simulink model "Suspension_shaker_rig_model"  (R2024b)
settings: Solver=VariableStepAuto  StartTime=0.0  StopTime=10  RelTol=1e-3
values from neighbouring files (symbols this model uses):
  a = 1.8    [Suspension_shaker_rig_model_parameters.m]
  A = 1.25    [Suspension_shaker_rig_model_parameters.m]
  a1f = -1e-5    (= -1e-05)    [Suspension_shaker_rig_model_parameters.m]
  a2f = 0.95    [Suspension_shaker_rig_model_parameters.m]
  b = L-a    (= 1.7)    [Suspension_shaker_rig_model_parameters.m]
  Bf = 0.0813    [Suspension_shaker_rig_model_parameters.m]
  Br = 0.0925    [Suspension_shaker_rig_model_parameters.m]
  cdf = 1400    [Suspension_shaker_rig_model_parameters.m]
  cdr = 1800    [Suspension_shaker_rig_model_parameters.m]
  Cf = 1.2947    [Suspension_shaker_rig_model_parameters.m]
  Cr = 1.2617    [Suspension_shaker_rig_model_parameters.m]
  Cz = 1.0    (= 1)    [Suspension_shaker_rig_model_parameters.m]
  Ef = -8.3966    [Suspension_shaker_rig_model_parameters.m]
  Er = -8.7012    [Suspension_shaker_rig_model_parameters.m]
  g = 9.81    [Suspension_shaker_rig_model_parameters.m]
  hrcf = 0.04    [Suspension_shaker_rig_model_parameters.m]
  hrcr = 0.06    [Suspension_shaker_rig_model_parameters.m]
  husmf = r    (= 0.375)    [Suspension_shaker_rig_model_parameters.m]
  husmr = r    (= 0.375)    [Suspension_shaker_rig_model_parameters.m]
  I = 3500    [Suspension_shaker_rig_model_parameters.m]
  Ixx = 300    [Suspension_shaker_rig_model_parameters.m]
  Iyy = 1350    [Suspension_shaker_rig_model_parameters.m]
  karbf = 5000    [Suspension_shaker_rig_model_parameters.m]
  karbr = 1000    [Suspension_shaker_rig_model_parameters.m]
  ksf = 67500    [Suspension_shaker_rig_model_parameters.m]
  ksr = 100000    [Suspension_shaker_rig_model_parameters.m]
  ktyre = 400000    [Suspension_shaker_rig_model_parameters.m]
  L = 3.5    [Suspension_shaker_rig_model_parameters.m]
  m = 850    [Suspension_shaker_rig_model_parameters.m]
  ms = m-(musf+musr)    (= 817.5)    [Suspension_shaker_rig_model_parameters.m]
  musf = 15.00    (= 15)    [Suspension_shaker_rig_model_parameters.m]
  musr = 17.50    (= 17.5)    [Suspension_shaker_rig_model_parameters.m]
  rho = 1.225    [Suspension_shaker_rig_model_parameters.m]
  tr = 1.85    [Suspension_shaker_rig_model_parameters.m]
  z0tfl = (0.5*ms*b/L+musf)*g/ktyre    (= 0.00523696339286)    [Suspension_shaker_rig_model_parameters.m]
  z0tfr = (0.5*ms*b/L+musf)*g/ktyre    (= 0.00523696339286)    [Suspension_shaker_rig_model_parameters.m]
  z0trl = (0.5*ms*a/L+musr)*g/ktyre    (= 0.00558469285714)    [Suspension_shaker_rig_model_parameters.m]
  z0trr = (0.5*ms*a/L+musr)*g/ktyre    (= 0.00558469285714)    [Suspension_shaker_rig_model_parameters.m]
libraries: aerolibconvert2 x5
settings Model: Creator=jayku  LastModifiedBy=jayku

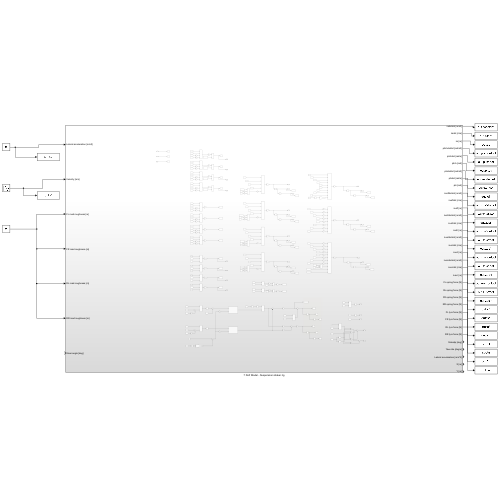
[thumbnail: Simulink's stored preview of the top-level diagram]
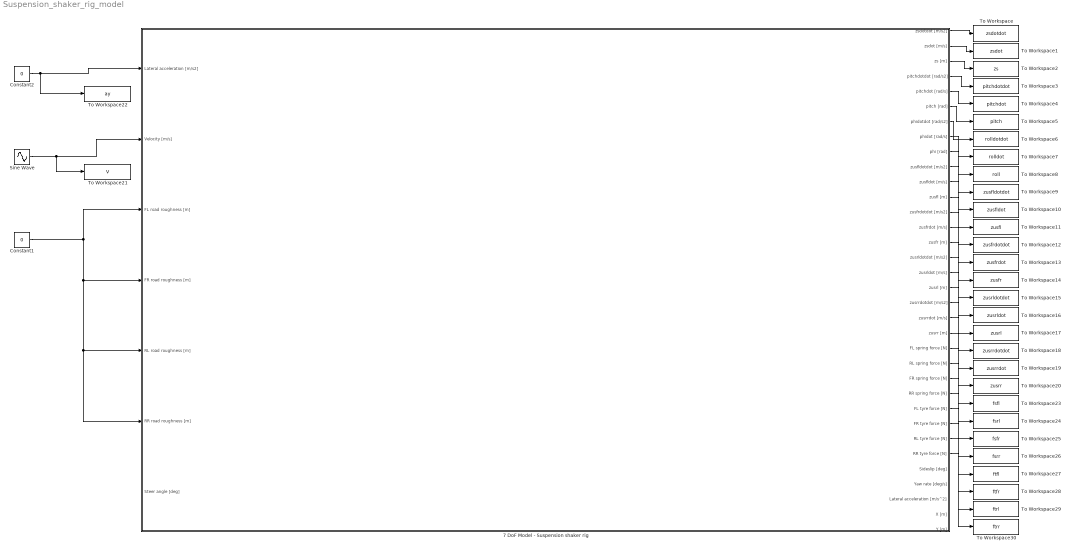
== system Suspension_shaker_rig_model ==
  7 DoF Model - Suspension shaker rig : Subsystem
  Constant1 : Constant  Value=0
  Constant2 : Constant  Value=0
  Sine Wave : Sin  Amplitude=0.01  Frequency=2*pi*1  SampleTime=0
  To Workspace : ToWorkspace  VariableName=zsdotdot  SaveFormat=Timeseries  SampleTime=-1
  To Workspace1 : ToWorkspace  VariableName=zsdot  SaveFormat=Timeseries  SampleTime=-1
  To Workspace10 : ToWorkspace  VariableName=zusfldot  SaveFormat=Timeseries  SampleTime=-1
  To Workspace11 : ToWorkspace  VariableName=zusfl  SaveFormat=Timeseries  SampleTime=-1
  To Workspace12 : ToWorkspace  VariableName=zusfrdotdot  SaveFormat=Timeseries  SampleTime=-1
  To Workspace13 : ToWorkspace  VariableName=zusfrdot  SaveFormat=Timeseries  SampleTime=-1
  To Workspace14 : ToWorkspace  VariableName=zusfr  SaveFormat=Timeseries  SampleTime=-1
  To Workspace15 : ToWorkspace  VariableName=zusrldotdot  SaveFormat=Timeseries  SampleTime=-1
  To Workspace16 : ToWorkspace  VariableName=zusrldot  SaveFormat=Timeseries  SampleTime=-1
  To Workspace17 : ToWorkspace  VariableName=zusrl  SaveFormat=Timeseries  SampleTime=-1
  To Workspace18 : ToWorkspace  VariableName=zusrrdotdot  SaveFormat=Timeseries  SampleTime=-1
  To Workspace19 : ToWorkspace  VariableName=zusrrdot  SaveFormat=Timeseries  SampleTime=-1
  To Workspace2 : ToWorkspace  VariableName=zs  SaveFormat=Timeseries  SampleTime=-1
  To Workspace20 : ToWorkspace  VariableName=zusrr  SaveFormat=Timeseries  SampleTime=-1
  To Workspace21 : ToWorkspace  VariableName=V  SaveFormat=Timeseries  SampleTime=-1
  To Workspace22 : ToWorkspace  VariableName=ay  SaveFormat=Timeseries  SampleTime=-1
  To Workspace23 : ToWorkspace  VariableName=fsfl  SaveFormat=Timeseries  SampleTime=-1
  To Workspace24 : ToWorkspace  VariableName=fsrl  SaveFormat=Timeseries  SampleTime=-1
  To Workspace25 : ToWorkspace  VariableName=fsfr  SaveFormat=Timeseries  SampleTime=-1
  To Workspace26 : ToWorkspace  VariableName=fsrr  SaveFormat=Timeseries  SampleTime=-1
  To Workspace27 : ToWorkspace  VariableName=ftfl  SaveFormat=Timeseries  SampleTime=-1
  To Workspace28 : ToWorkspace  VariableName=ftfr  SaveFormat=Timeseries  SampleTime=-1
  To Workspace29 : ToWorkspace  VariableName=ftrl  SaveFormat=Timeseries  SampleTime=-1
  To Workspace3 : ToWorkspace  VariableName=pitchdotdot  SaveFormat=Timeseries  SampleTime=-1
  To Workspace30 : ToWorkspace  VariableName=ftrr  SaveFormat=Timeseries  SampleTime=-1
  To Workspace4 : ToWorkspace  VariableName=pitchdot  SaveFormat=Timeseries  SampleTime=-1
  To Workspace5 : ToWorkspace  VariableName=pitch  SaveFormat=Timeseries  SampleTime=-1
  To Workspace6 : ToWorkspace  VariableName=rolldotdot  SaveFormat=Timeseries  SampleTime=-1
  To Workspace7 : ToWorkspace  VariableName=rolldot  SaveFormat=Timeseries  SampleTime=-1
  To Workspace8 : ToWorkspace  VariableName=roll  SaveFormat=Timeseries  SampleTime=-1
  To Workspace9 : ToWorkspace  VariableName=zusfldotdot  SaveFormat=Timeseries  SampleTime=-1
  wires:
  7 DoF Model - Suspension shaker rig/1(zsdotdot [m/s2]) -> To Workspace/1
  7 DoF Model - Suspension shaker rig/2(zsdot [m/s]) -> To Workspace1/1
  7 DoF Model - Suspension shaker rig/3(zs [m]) -> To Workspace2/1
  7 DoF Model - Suspension shaker rig/4(pitchdotdot [rad/s2]) -> To Workspace3/1
  7 DoF Model - Suspension shaker rig/5(pitchdot [rad/s]) -> To Workspace4/1
  7 DoF Model - Suspension shaker rig/6(pitch [rad]) -> To Workspace5/1
  7 DoF Model - Suspension shaker rig/7(phidotdot [rad/s2]) -> To Workspace6/1
  7 DoF Model - Suspension shaker rig/8(phidot [rad/s]) -> To Workspace7/1
  7 DoF Model - Suspension shaker rig/9(phi [rad]) -> To Workspace8/1
  7 DoF Model - Suspension shaker rig/10(zusfldotdot [m/s2]) -> To Workspace9/1
  7 DoF Model - Suspension shaker rig/11(zusfldot [m/s]) -> To Workspace10/1
  7 DoF Model - Suspension shaker rig/12(zusfl [m]) -> To Workspace11/1
  7 DoF Model - Suspension shaker rig/13(zusfrdotdot [m/s2]) -> To Workspace12/1
  7 DoF Model - Suspension shaker rig/14(zusfrdot [m/s]) -> To Workspace13/1
  7 DoF Model - Suspension shaker rig/15(zusfr [m]) -> To Workspace14/1
  7 DoF Model - Suspension shaker rig/16(zusrldotdot [m/s2]) -> To Workspace15/1
  7 DoF Model - Suspension shaker rig/17(zusrldot [m/s]) -> To Workspace16/1
  7 DoF Model - Suspension shaker rig/18(zusrl [m]) -> To Workspace17/1
  7 DoF Model - Suspension shaker rig/19(zusrrdotdot [m/s2]) -> To Workspace18/1
  7 DoF Model - Suspension shaker rig/20(zusrrdot [m/s]) -> To Workspace19/1
  7 DoF Model - Suspension shaker rig/21(zusrr [m]) -> To Workspace20/1
  Constant2/1 -> 7 DoF Model - Suspension shaker rig/1(Lateral acceleration [m/s2]), To Workspace22/1
  Sine Wave/1 -> 7 DoF Model - Suspension shaker rig/2(Velocity [m/s]), To Workspace21/1
  7 DoF Model - Suspension shaker rig/22(FL spring force [N]) -> To Workspace23/1
  7 DoF Model - Suspension shaker rig/23(RL spring force [N]) -> To Workspace24/1
  7 DoF Model - Suspension shaker rig/24(FR spring force [N]) -> To Workspace25/1
  7 DoF Model - Suspension shaker rig/25(RR spring force [N]) -> To Workspace26/1
  7 DoF Model - Suspension shaker rig/26(FL tyre force [N]) -> To Workspace27/1
  7 DoF Model - Suspension shaker rig/27(FR tyre force [N]) -> To Workspace28/1
  7 DoF Model - Suspension shaker rig/28(RL tyre force [N]) -> To Workspace29/1
  7 DoF Model - Suspension shaker rig/29(RR tyre force [N]) -> To Workspace30/1
  Constant1/1 -> 7 DoF Model - Suspension shaker rig/5(RL road roughness [m]), 7 DoF Model - Suspension shaker rig/6(RR road roughness [m]), 7 DoF Model - Suspension shaker rig/4(FR road roughness [m]), 7 DoF Model - Suspension shaker rig/3(FL road roughness [m])

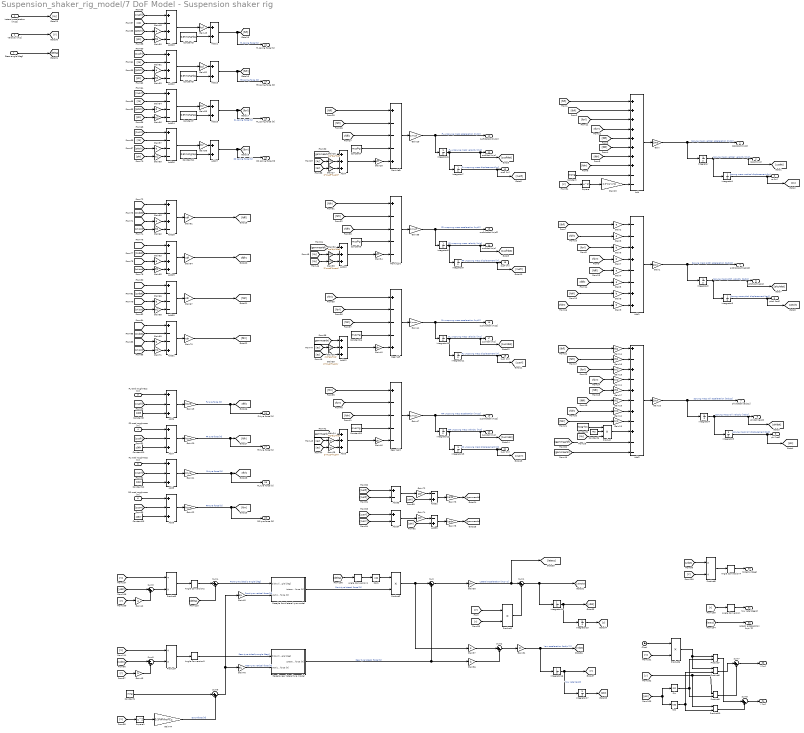
== system Suspension_shaker_rig_model/7 DoF Model - Suspension shaker rig ==
  Lateral acceleration [m/s2] : Inport
  Velocity [m/s] : Inport  Port=2
  FL road roughness [m] : Inport  Port=3
  FR road roughness [m] : Inport  Port=4
  RL road roughness [m] : Inport  Port=5
  RR road roughness [m] : Inport  Port=6
  Steer angle [deg] : Inport  Port=7
  Add : Sum  Inputs=++++++++--
  Add1 : Sum  Inputs=--++--++
  Add{3..4,10,12} (4 alike) : Sum  Inputs=+++
  Add2 : Sum  Inputs=+-+-+-+-+--
  Add20 : Sum  Inputs=+-+-
  Add{21,23,25,27} (4 alike) : Sum
  Add22 : Sum  Inputs=+-+-
  Add24 : Sum  Inputs=+---
  Add26 : Sum  Inputs=+---
  Add28 : Sum  Inputs=+-+-
  Add29 : Sum  Inputs=+-++
  Add30 : Sum  Inputs=+---
  Add31 : Sum  Inputs=+--+
  Add32 : Sum  Inputs=-+
  Add33 : Sum  Inputs=+-
  Add34 : Sum  Inputs=+-
  Add35 : Sum  Inputs=-+
  Add{6..9} (4 alike) : Sum  Inputs=+-+
  Angle Conversion{,2..4} (4 alike) : aerolibconvert2/Angle Conversion  IU=rad  OU=deg
  Angle Conversion1 : aerolibconvert2/Angle Conversion  IU=deg  OU=rad
  Clock : Clock
  Constant : Constant  Value=ms*g
  Constant1 : Constant  Value=m*g
  Constant10 : Constant  Value=z0tfr
  Constant11 : Constant  Value=0.5*ms*g*a/L
  Constant12 : Constant  Value=z0trl
  Constant13 : Constant  Value=z0trr
  Constant16 : Constant  Value=musr*g
  Constant2 : Constant  Value=hcog-hrc
  Constant20 : Constant  Value=musr*g
  Constant3 : Constant  Value=0.5*ms*g*b/L
  Constant4 : Constant  Value=musf*g
  Constant5 : Constant  Value=0.5*ms*g*b/L
  Constant6 : Constant  Value=ms
  Constant7 : Constant  Value=0.5*ms*g*a/L
  Constant8 : Constant  Value=z0tfl
  Constant9 : Constant  Value=musf*g
  Cos : Trigonometry  Operator=cos
  Cos1 : Trigonometry  Operator=cos
  Front left : Sum  Inputs=+---+
  Front right : Sum  Inputs=+----
  Gain : Gain  Gain=1/ms
  Gain1 : Gain  Gain=1/Iyy
  Gain10 : Gain  Gain=1/Ixx
  Gain{11..13,15,56,59,68,71} (8 alike) : Gain  Gain=tr/2
  Gain{14,16..18,50,53,62,65} (8 alike) : Gain  Gain=tf/2
  Gain{19..22} (4 alike) : Gain  Gain=ktyre
  Gain{2..5,37,42,48,51,60,63} (10 alike) : Gain  Gain=a
  Gain23 : Gain  Gain=0.5*rho*A*Cz
  Gain24 : Gain  Gain=ms*a/L*hrcr
  Gain25 : Gain  Gain=2*musr*husmr
  Gain26 : Gain  Gain=ms*b/L*hrcf
  Gain27 : Gain  Gain=2*musf*husmf
  Gain28 : Gain  Gain=1/tf
  Gain29 : Gain  Gain=1/musf
  Gain30 : Gain  Gain=1/m
  Gain31 : Gain  Gain=1/I
  Gain32 : Gain  Gain=ms*b/L*hrcf
  Gain33 : Gain  Gain=2*musf*husmf
  Gain34 : Gain  Gain=1/tf
  Gain35 : Gain  Gain=1/musf
  Gain{6..9,36,43,54,57,66,69} (10 alike) : Gain  Gain=b
  Gain38 : Gain  Gain=ms*a/L*hrcr
  Gain39 : Gain  Gain=2*musr*husmr
  Gain40 : Gain  Gain=1/tr
  Gain41 : Gain  Gain=1/musr
  Gain44 : Gain  Gain=0.5*A*rho*Cz
  Gain45 : Gain  Gain=b/L
  Gain46 : Gain  Gain=1/tr
  Gain47 : Gain  Gain=1/musr
  Gain49 : Gain  Gain=ksf
  Gain52 : Gain  Gain=ksf
  Gain55 : Gain  Gain=ksr
  Gain58 : Gain  Gain=ksr
  Gain61 : Gain  Gain=cdf
  Gain64 : Gain  Gain=cdf
  Gain67 : Gain  Gain=cdr
  Gain70 : Gain  Gain=cdr
  Gain72 : Gain  Gain=1/tf
  Gain73 : Gain  Gain=karbf
  Gain74 : Gain  Gain=1/tr
  Gain75 : Gain  Gain=karbr
  Gain76 : Gain  Gain=a/L
  Integrator{,1..17} (18 alike) : Integrator
  Pacejka front lateral tyre model : Subsystem
  Pacejka rear lateral tyre model : Subsystem
  Product : Product  Inputs=***
  Product{1..2,6..10} (7 alike) : Product
  Product3 : Product  Inputs=/*
  Product4 : Product  Inputs=/*
  Product5 : Product  Inputs=*/
  Rear left : Sum  Inputs=+---+
  Rear right : Sum  Inputs=+----
  Sin : Trigonometry
  Square : Math  Operator=square
  Square1 : Math  Operator=square
  Sum{,3,6,8} (4 alike) : Sum  Inputs=|++
  Sum{1..2,4..5,7} (5 alike) : Sum  Inputs=|+-
  zsdotdot [m/s2] : Outport
  zsdot [m/s] : Outport  Port=2
  zs [m] : Outport  Port=3
  pitchdotdot [rad/s2] : Outport  Port=4
  pitchdot [rad/s] : Outport  Port=5
  pitch [rad] : Outport  Port=6
  phidotdot [rad/s2] : Outport  Port=7
  phidot [rad/s] : Outport  Port=8
  phi [rad] : Outport  Port=9
  zusfldotdot [m/s2] : Outport  Port=10
  zusfldot [m/s] : Outport  Port=11
  zusfl [m] : Outport  Port=12
  zusfrdotdot [m/s2] : Outport  Port=13
  zusfrdot [m/s] : Outport  Port=14
  zusfr [m] : Outport  Port=15
  zusrldotdot [m/s2] : Outport  Port=16
  zusrldot [m/s] : Outport  Port=17
  zusrl [m] : Outport  Port=18
  zusrrdotdot [m/s2] : Outport  Port=19
  zusrrdot [m/s] : Outport  Port=20
  zusrr [m] : Outport  Port=21
  FL spring force [N] : Outport  Port=22
  RL spring force [N] : Outport  Port=23
  FR spring force [N] : Outport  Port=24
  RR spring force [N] : Outport  Port=25
  FL tyre force [N] : Outport  Port=26
  FR tyre force [N] : Outport  Port=27
  RL tyre force [N] : Outport  Port=28
  RR tyre force [N] : Outport  Port=29
  Sideslip [deg] : Outport  Port=30
  Yaw rate [deg/s] : Outport  Port=31
  Lateral acceleration [m/s^2] : Outport  Port=32
  X [m] : Outport  Port=33
  Y [m] : Outport  Port=34
  wires:
  Integrator1/1 -> [zs], zs [m]/1  "Sprung mass vertical displacement [m]"
  Add/1 -> Gain/1
  [fsrr] -> Add/4
  [fsfl] -> Add/1
  [fsrl] -> Add/3
  Integrator/1 -> [zsdot], zsdot [m/s]/1, Integrator1/1  "Sprung mass vertical velocity [m/s]"
  [fsfr] -> Add/2
  [fdfl] -> Add/5
  [fdfr] -> Add/6
  [fdrl] -> Add/7
  [fdrr] -> Add/8
  Constant/1 -> Add/9
  [V] -> Square/1
  Gain/1 -> zsdotdot [m/s2]/1, Integrator/1  "Sprung mass vertical acceleration [m/s2]"
  [fdrl] -> Gain8/1
  [fdfl] -> Gain4/1
  Add1/1 -> Gain1/1
  Integrator3/1 -> [pitch], pitch [rad]/1  "Sprung mass pitch displacement [rad]"
  [fdrr] -> Gain9/1
  [fsfl] -> Gain2/1
  Integrator2/1 -> [pitchdot], pitchdot [rad/s]/1, Integrator3/1  "Sprung mass pitch velocity [rad/s]"
  [fsfr] -> Gain3/1
  Gain1/1 -> pitchdotdot [rad/s2]/1, Integrator2/1  "Sprung mass pitch acceleration [rad/s2]"
  [fsrl] -> Gain6/1
  [fsrr] -> Gain7/1
  [fdfr] -> Gain5/1
  Gain2/1 -> Add1/1
  Gain3/1 -> Add1/2
  Gain4/1 -> Add1/5
  Gain5/1 -> Add1/6
  Gain6/1 -> Add1/3
  Gain7/1 -> Add1/4
  Gain8/1 -> Add1/7
  Gain9/1 -> Add1/8
  Gain13/1 -> Add2/8
  Gain12/1 -> Add2/7
  Gain11/1 -> Add2/4
  Gain15/1 -> Add2/3
  [fdfr] -> Gain18/1
  [fdfl] -> Gain17/1
  [fsfr] -> Gain16/1
  [fsfl] -> Gain14/1
  [fsrr] -> Gain11/1
  [fsrl] -> Gain15/1
  Gain10/1 -> phidotdot [rad/s2]/1, Integrator4/1  "Sprung mass roll acceleration [rad/s2]"
  Integrator4/1 -> Integrator5/1, [phidot], phidot [rad/s]/1  "Sprung mass roll velocity [rad/s]"
  [fdrr] -> Gain13/1
  Integrator5/1 -> [phi], phi [rad]/1  "Sprung mass roll displacement [rad]"
  Add2/1 -> Gain10/1
  [fdrl] -> Gain12/1
  Gain14/1 -> Add2/1
  Gain16/1 -> Add2/2
  Gain17/1 -> Add2/5
  Gain18/1 -> Add2/6
  Constant4/1 -> Front left/4
  [fdfl] -> Front left/3
  [fsfl] -> Front left/2
  [ftfl] -> Front left/1
  [gammaarbf] -> Add4/1
  Gain26/1 -> Add4/2
  [ay] -> Gain26/1
  Gain27/1 -> Add4/3
  [ay] -> Gain27/1
  Gain28/1 -> Front left/5
  Add4/1 -> Gain28/1
  Front left/1 -> Gain29/1
  Integrator7/1 -> zusfl [m]/1, [zusfl]  "FL unsprung mass displacement [m]"
  Integrator6/1 -> zusfldot [m/s]/1, [zusfldot], Integrator7/1  "FL unsprung mass velocity [m/s]"
  Gain29/1 -> Integrator6/1, zusfldotdot [m/s2]/1  "FL unsprung mass acceleration [m/s2]"
  Gain35/1 -> zusfrdotdot [m/s2]/1, Integrator8/1  "FR unsprung mass acceleration [m/s2]"
  Integrator8/1 -> Integrator9/1, [zusfrdot], zusfrdot [m/s]/1  "FR unsprung mass velocity [m/s]"
  Integrator9/1 -> [zusfr], zusfr [m]/1  "FR unsprung mass displacement [m]"
  Front right/1 -> Gain35/1
  Add10/1 -> Gain34/1
  Gain34/1 -> Front right/5
  Gain33/1 -> Add10/3
  Gain32/1 -> Add10/2
  [gammaarbf] -> Add10/1
  [ftfr] -> Front right/1
  [fsfr] -> Front right/2
  [fdfr] -> Front right/3
  Constant9/1 -> Front right/4
  Constant16/1 -> Rear left/4
  [fdrl] -> Rear left/3
  [fsrl] -> Rear left/2
  [ftrl] -> Rear left/1
  [gammaarbr] -> Add12/1
  Gain38/1 -> Add12/2
  Gain39/1 -> Add12/3
  Gain40/1 -> Rear left/5
  Add12/1 -> Gain40/1
  Rear left/1 -> Gain41/1
  Integrator11/1 -> zusrl [m]/1, [zusrl]  "RL unsprung mass displacement [m]"
  Integrator10/1 -> zusrldot [m/s]/1, [zusrldot], Integrator11/1  "RL unsprung mass velocity [m/s]"
  Gain41/1 -> Integrator10/1, zusrldotdot [m/s2]/1  "RL unsprung mass acceleration [m/s2]"
  Gain47/1 -> zusrrdotdot [m/s2]/1, Integrator12/1  "RR unsprung mass acceleration [m/s2]"
  Integrator12/1 -> Integrator13/1, [zusrrdot], zusrrdot [m/s]/1  "RR unsprung mass velocity [m/s]"
  Integrator13/1 -> [zusrr], zusrr [m]/1  "RR unsprung mass displacement [m]"
  Rear right/1 -> Gain47/1
  Add3/1 -> Gain46/1
  Gain46/1 -> Rear right/5
  [gammaarbr] -> Add3/1
  [ftrr] -> Rear right/1
  [fsrr] -> Rear right/2
  [fdrr] -> Rear right/3
  Constant20/1 -> Rear right/4
  Add21/1 -> FL spring force [N]/1, [fsfl]  "FL spring force [N]"
  Gain48/1 -> Add20/3
  Gain49/1 -> Add21/1
  [zs] -> Add20/2
  [zusfl] -> Add20/1
  Add20/1 -> Gain49/1
  [pitch] -> Gain48/1
  Constant3/1 -> Add21/2
  Gain50/1 -> Add20/4
  [phi] -> Gain50/1
  [phi] -> Gain53/1
  Gain53/1 -> Add22/4
  Constant5/1 -> Add23/2
  [pitch] -> Gain51/1
  Add22/1 -> Gain52/1
  [zusfr] -> Add22/1
  [zs] -> Add22/2
  Gain52/1 -> Add23/1
  Gain51/1 -> Add22/3
  Add23/1 -> FR spring force [N]/1, [fsfr]  "FR spring force [N]"
  Add25/1 -> RL spring force [N]/1, [fsrl]  "RL spring force [N]"
  Gain54/1 -> Add24/3
  Gain55/1 -> Add25/1
  [zs] -> Add24/2
  [zusrl] -> Add24/1
  Add24/1 -> Gain55/1
  [pitch] -> Gain54/1
  Constant7/1 -> Add25/2
  Gain56/1 -> Add24/4
  [phi] -> Gain56/1
  [phi] -> Gain59/1
  Gain59/1 -> Add26/4
  Constant11/1 -> Add27/2
  [pitch] -> Gain57/1
  Add26/1 -> Gain58/1
  [zusrr] -> Add26/1
  [zs] -> Add26/2
  Gain58/1 -> Add27/1
  Gain57/1 -> Add26/3
  Add27/1 -> RR spring force [N]/1, [fsrr]  "RR spring force [N]"
  Gain60/1 -> Add28/3
  [zsdot] -> Add28/2
  [zusfldot] -> Add28/1
  Add28/1 -> Gain61/1
  Gain61/1 -> [fdfl]
  [pitchdot] -> Gain60/1
  [phidot] -> Gain62/1
  Gain62/1 -> Add28/4
  Gain65/1 -> Add29/4
  [phidot] -> Gain65/1
  [pitchdot] -> Gain63/1
  Gain64/1 -> [fdfr]
  Add29/1 -> Gain64/1
  [zusfrdot] -> Add29/1
  [zsdot] -> Add29/2
  Gain63/1 -> Add29/3
  Gain66/1 -> Add30/3
  [zsdot] -> Add30/2
  [zusrldot] -> Add30/1
  Add30/1 -> Gain67/1
  Gain67/1 -> [fdrl]
  [pitchdot] -> Gain66/1
  [phidot] -> Gain68/1
  Gain68/1 -> Add30/4
  Gain71/1 -> Add31/4
  [phidot] -> Gain71/1
  [pitchdot] -> Gain69/1
  Gain70/1 -> [fdrr]
  Add31/1 -> Gain70/1
  [zusrrdot] -> Add31/1
  [zsdot] -> Add31/2
  Gain69/1 -> Add31/3
  Lateral acceleration [m/s2]/1 -> [ay]
  Add33/1 -> Gain72/1
  [phi] -> Add32/2
  Gain72/1 -> Add32/1
  [zusfl] -> Add33/1
  Add32/1 -> Gain73/1
  [zusfr] -> Add33/2
  Gain73/1 -> [gammaarbf]
  [phi] -> Add35/2
  Gain74/1 -> Add35/1
  Add34/1 -> Gain74/1
  [zusrl] -> Add34/1
  Add35/1 -> Gain75/1
  [zusrr] -> Add34/2
  Gain75/1 -> [gammaarbr]
  Gain24/1 -> Add3/2
  Gain25/1 -> Add3/3
  [ay] -> Gain24/1
  [ay] -> Gain25/1
  [ay] -> Gain32/1
  [ay] -> Gain33/1
  [ay] -> Gain38/1
  [ay] -> Gain39/1
  [gammaarbf] -> Add2/10
  [gammaarbr] -> Add2/11
  Constant2/1 -> Product/1
  Constant6/1 -> Product/2
  [ay] -> Product/3
  Product/1 -> Add2/9
  Constant8/1 -> Add6/3
  FL road roughness [m]/1 -> Add6/1
  Add6/1 -> Gain19/1
  Gain19/1 -> FL tyre force [N]/1, [ftfl]  "FL tyre force [N]"
  [zusfl] -> Add6/2
  [zusfr] -> Add7/2
  Gain20/1 -> FR tyre force [N]/1, [ftfr]  "FR tyre force [N]"
  Add7/1 -> Gain20/1
  FR road roughness [m]/1 -> Add7/1
  Constant10/1 -> Add7/3
  Constant12/1 -> Add8/3
  RL road roughness [m]/1 -> Add8/1
  Add8/1 -> Gain21/1
  Gain21/1 -> RL tyre force [N]/1, [ftrl]  "RL tyre force [N]"
  [zusrl] -> Add8/2
  [zusrr] -> Add9/2
  Gain22/1 -> RR tyre force [N]/1, [ftrr]  "RR tyre force [N]"
  Add9/1 -> Gain22/1
  RR road roughness [m]/1 -> Add9/1
  Constant13/1 -> Add9/3
  Gain23/1 -> Add/10
  Velocity [m/s]/1 -> [V]
  Square/1 -> Gain23/1
  Angle Conversion/1 -> Yaw rate [deg/s]/1
  [V] -> Product4/1
  [ydot] -> Product5/1
  Gain43/1 -> Sum5/2
  Square1/1 -> Gain44/1
  [ydot] -> Sum3/1
  Sum7/1 -> X [m]/1
  Gain76/1 -> Pacejka rear lateral tyre model/2(Vertical force [N])  "Rear tyre vertical force [N]"
  Sum5/1 -> Product4/2
  Integrator15/1 -> [y]
  Clock/1 -> Product6/1
  [r] -> Angle Conversion/1
  Sum2/1 -> Gain31/1
  Gain36/1 -> Sum2/2
  Integrator17/1 -> [psi]
  Cos/1 -> Product8/2, Product10/2
  [latacc] -> Lateral acceleration [m/s^2]/1
  [y] -> Product10/1, Product9/1
  [r] -> Gain42/1
  [V] -> Product1/1
  [V] -> Product3/1
  [V] -> Product6/2
  Angle Conversion3/1 -> Pacejka rear lateral tyre model/1(Side slip angle [deg])  "Rear tyre sideslip angle [deg]"
  Product3/1 -> Angle Conversion2/1
  [r] -> Gain43/1
  Product10/1 -> Sum8/2
  [r] -> Product1/2
  [delta] -> Sum4/2
  Sum4/1 -> Pacejka front lateral tyre model/1(Side slip angle [deg])  "Front tyre sideslip angle [deg]"
  Integrator16/1 -> [r], Integrator17/1  "Yaw rate [rad/s]"
  Product4/1 -> Angle Conversion3/1
  Sum/1 -> Gain30/1
  Cos1/1 -> Product2/1
  Product1/1 -> Sum1/2
  Sum8/1 -> Y [m]/1
  Angle Conversion4/1 -> Sideslip [deg]/1
  [psi] -> Sin/1, Cos/1
  [delta] -> Angle Conversion1/1
  Gain45/1 -> Pacejka front lateral tyre model/2(Vertical force [N])  "Front tyre vertical force [N]"
  Product2/1 -> Gain37/1, Sum/1
  Gain37/1 -> Sum2/1
  Product7/1 -> Sum8/1
  Angle Conversion2/1 -> Sum4/1
  Gain42/1 -> Sum3/2
  Sum1/1 -> Integrator14/1, [ydotdot]
  Product5/1 -> Angle Conversion4/1
  Product6/1 -> Product8/1, Product7/1
  Gain30/1 -> [latacc], Sum1/1  "Lateral acceleration [m/s^2]"
  Pacejka front lateral tyre model/1(Lateral force [N]) -> Product2/2  "Front tyre lateral force [N]"
  Steer angle [deg]/1 -> [delta]
  Constant1/1 -> Sum6/1
  [ydot] -> Sum5/1
  Gain44/1 -> Sum6/2  "Downforce [N]"
  Product8/1 -> Sum7/1
  [V] -> Square1/1
  Integrator14/1 -> Integrator15/1, [ydot]
  [V] -> Product5/2
  Product9/1 -> Sum7/2
  Sin/1 -> Product7/2, Product9/2
  Angle Conversion1/1 -> Cos1/1
  Sum3/1 -> Product3/2
  Pacejka rear lateral tyre model/1(Lateral force [N]) -> Gain36/1, Sum/2  "Rear tyre lateral force [N]"
  Sum6/1 -> Gain45/1, Gain76/1
  Gain31/1 -> [rdot], Integrator16/1  "Yaw acceleration [rad/s^2]"

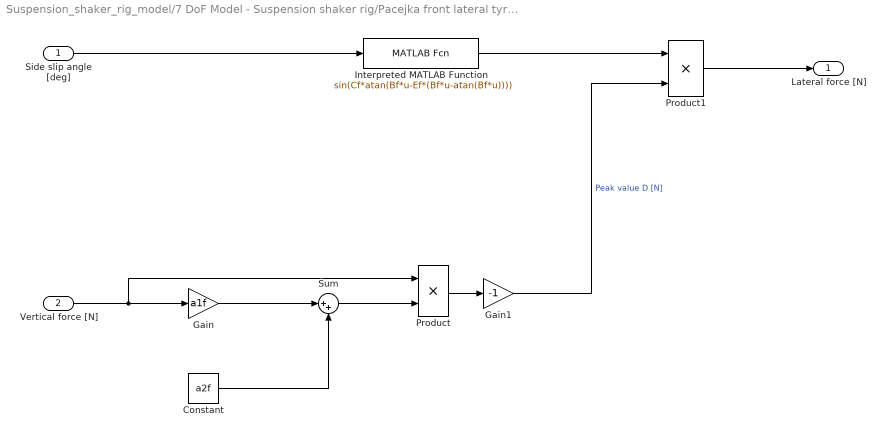
== system Suspension_shaker_rig_model/7 DoF Model - Suspension shaker rig/Pacejka front lateral tyre model ==
  Side slip angle [deg] : Inport
  Vertical force [N] : Inport  Port=2
  Constant : Constant  Value=a2f
  Gain : Gain  Gain=a1f
  Gain1 : Gain  Gain=-1
  Interpreted MATLAB Function : MATLABFcn  MATLABFcn=sin(Cf*atan(Bf*u-Ef*(Bf*u-atan(Bf*u))))
  Product : Product
  Product1 : Product
  Sum : Sum  Inputs=|++
  Lateral force [N] : Outport
  wires:
  Side slip angle [deg]/1 -> Interpreted MATLAB Function/1
  Vertical force [N]/1 -> Product/1, Gain/1
  Gain/1 -> Sum/1
  Constant/1 -> Sum/2
  Sum/1 -> Product/2
  Product/1 -> Gain1/1
  Gain1/1 -> Product1/2  "Peak value D [N]"
  Interpreted MATLAB Function/1 -> Product1/1
  Product1/1 -> Lateral force [N]/1

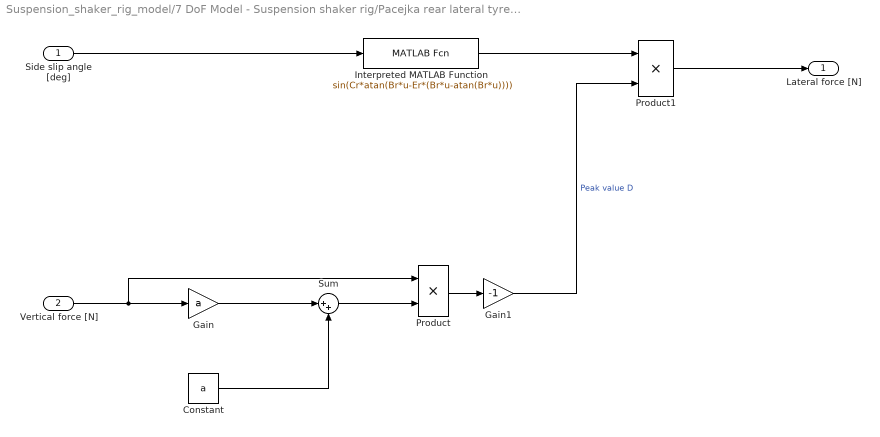
== system Suspension_shaker_rig_model/7 DoF Model - Suspension shaker rig/Pacejka rear lateral tyre model ==
  Side slip angle [deg] : Inport
  Vertical force [N] : Inport  Port=2
  Constant : Constant  Value=a
  Gain : Gain  Gain=a
  Gain1 : Gain  Gain=-1
  Interpreted MATLAB Function : MATLABFcn  MATLABFcn=sin(Cr*atan(Br*u-Er*(Br*u-atan(Br*u))))
  Product : Product
  Product1 : Product
  Sum : Sum  Inputs=|++
  Lateral force [N] : Outport
  wires:
  Side slip angle [deg]/1 -> Interpreted MATLAB Function/1
  Vertical force [N]/1 -> Product/1, Gain/1
  Gain/1 -> Sum/1
  Constant/1 -> Sum/2
  Sum/1 -> Product/2
  Product/1 -> Gain1/1
  Gain1/1 -> Product1/2  "Peak value D"
  Interpreted MATLAB Function/1 -> Product1/1
  Product1/1 -> Lateral force [N]/1
